simulink model "q4"  (R2017a)
settings: Solver=VariableStepAuto  StartTime=0.0  StopTime=4.0  FixedStep=T  RelTol=1e-3
libraries: cstblocks x2
settings Model: Creator=arthur  LastModifiedBy=arthur

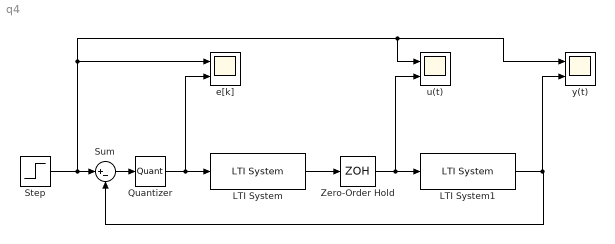
== system q4 ==
  LTI System : cstblocks/LTI System  sys=Gc2_z  IC=[]
  LTI System1 : cstblocks/LTI System  sys=G_s  IC=[]
  Quantizer : Quantizer  QuantizationInterval=T
  Step : Step  Time=0
  Sum : Sum  Inputs=|+-
  Zero-Order Hold : ZeroOrderHold  SampleTime=-1
  e[k] : Scope  NumInputPorts=2
  u(t) : Scope  NumInputPorts=2
  y(t) : Scope  NumInputPorts=2
  wires:
  Step/1 -> y(t)/1, u(t)/1, e[k]/1, Sum/1
  Zero-Order Hold/1 -> u(t)/2, LTI System1/1
  LTI System/1 -> Zero-Order Hold/1
  LTI System1/1 -> y(t)/2, Sum/2
  Sum/1 -> Quantizer/1
  Quantizer/1 -> e[k]/2, LTI System/1
